simulink model "shift_register"  (R2020a)
settings: Solver=VariableStepAuto  StartTime=0.0  StopTime=10  RelTol=1e-3
libraries: simulink_extras x5
settings Model: EnablePacing=on  PacingRate=0.280000  Creator=F1  LastModifiedBy=F1
settings OptimizationCC: BooleanDataType=off

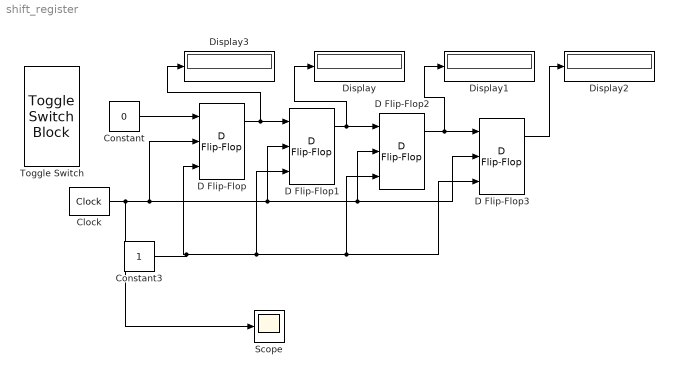
== system shift_register ==
  Clock : simulink_extras/Flip Flops/Clock  period=2
  Constant : Constant  Value=0
  Constant3 : Constant
  D Flip-Flop{,1..3} (4 alike) : simulink_extras/Flip Flops/D Flip-Flop
  Display{,1..3} (4 alike) : Display
  Scope : Scope
  Toggle Switch : ToggleSwitchBlock
      settings: Values={{'Off', 'On'}, [0 1]}
  wires:
  D Flip-Flop2/1 -> Display1/1, D Flip-Flop3/1
  D Flip-Flop1/1 -> D Flip-Flop2/1, Display/1
  D Flip-Flop/1 -> Display3/1, D Flip-Flop1/1
  Clock/1 -> Scope/1, D Flip-Flop3/2, D Flip-Flop2/2, D Flip-Flop1/2, D Flip-Flop/2
  Constant/1 -> D Flip-Flop/1
  D Flip-Flop3/1 -> Display2/1
  Constant3/1 -> D Flip-Flop/3, D Flip-Flop3/3, D Flip-Flop2/3, D Flip-Flop1/3
